simulink model "BDA_DynamicModel_v3"  (R2021b)
settings: Solver=ode23t  StartTime=0.0  StopTime=15  FixedStep=0.000001  MaxStep=1e-5  MinStep=1e-7  RelTol=1e-3
undefined symbols (not defined in the file or in its folder): X, Y, Z
libraries: sm_lib x47, nesl_utility x7
(part 3 of 5)

== matlab function BDA_DynamicModel_v3/Planta/Dinámica Directa/h ==
  data: dq1 input; h output; dq2 input; dq3 input; dq4 input; dq5 input; dq6 input; q1 input; q2 input; q3 input; q4 input; q5 input; q6 input
function h = h(dq1,dq2,dq3,dq4,dq5,dq6,q1,q2,q3,q4,q5,q6)
%#codegen

%    This function was generated by the Symbolic Math Toolbox version 9.0.
%    28-Nov-2021 14:58:02

t2 = cos(q1);
t3 = cos(q2);
t4 = cos(q4);
t5 = cos(q5);
t6 = cos(q6);
t7 = sin(q1);
t8 = sin(q2);
t9 = sin(q4);
t10 = sin(q5);
t11 = sin(q6);
t12 = dq1+dq2;
t14 = dq5.*(3.0./5.0e+2);
t22 = dq3.*5.110348748545983e-1;
t26 = dq3.*8.595599785252598e-1;
t27 = dq1.*2.038587e-2;
t28 = dq2.*2.038587e-2;
t30 = dq4.*2.889644e-2;
t31 = 9.007199254740992e+15;
t33 = dq6.*7.26735e-3;
t34 = dq5.*1.08769e-2;
t52 = dq3.*1.705747536335924e-3;
t55 = dq3.*2.869065083120968e-3;
t56 = dq3.*1.476708859914341e-2;
t58 = dq5.*6.1855407534e-5;
t59 = dq4.*6.678441185616e-4;
t60 = dq5.*1.35652563578e-4;
t61 = dq6.*1.33637554986e-4;
t62 = dq4.*1.688944904408e-4;
t63 = dq6.*7.26350557185e-5;
t65 = dq5.*7.0482312e-7;
t67 = dq4.*1.869599668e-7;
t88 = dq3.*1.749264567482926e-5;
t96 = dq3.*2.94226067152155e-5;
t97 = dq3.*1.573543573532208e-5;
t101 = dq3.*2.646698193853677e-5;
t102 = dq3.*4.515804245053758e-5;
t105 = dq3.*3.412916355515067e-4;
t106 = dq3.*8.631097478604537e-5;
t107 = dq4.*6.634286610512106e-7;
t108 = dq5.*7.314371377091851e-7;
t110 = dq6.*3.387428925624357e-6;
t111 = dq6.*1.745966317740249e-6;
t112 = dq6.*1.245668607194124e-6;
t113 = dq3.*9.554306323645785e-8;
t115 = dq5.*4.0082304082032e-9;
t116 = dq4.*2.626213073993121e-5;
t117 = dq4.*4.320951447093552e-9;
t118 = dq4.*1.092747353151976e-9;
t119 = dq5.*2.261852897508832e-6;
t120 = dq5.*5.918087154269792e-7;
t122 = dq5.*1.87902861198544e-8;
t124 = dq4.*2.3264974053944e-5;
t129 = dq3.*5.321009981904056e-7;
t135 = dq3.*4.369754608674261e-7;
t141 = dq3.*4.553682647545594e-7;
t142 = dq3.*3.390351827752591e-7;
t145 = dq3.*7.349921428868027e-7;
t153 = dq3.*1.342086469609585e-5;
t154 = dq3.*2.208156882018249e-9;
t155 = dq3.*5.584320068657135e-10;
t166 = dq3.*1.188921310415275e-5;
t13 = t12.^2;
t15 = t2.*t3.*(9.81e+2./1.0e+2);
t16 = t2.*t8.*(9.81e+2./1.0e+2);
t17 = t3.*t7.*(9.81e+2./1.0e+2);
t18 = t7.*t8.*(9.81e+2./1.0e+2);
t20 = t3.*1.051339e-1;
t21 = t8.*1.051339e-1;
t23 = t5.*5.110348748545983e-1;
t25 = t10.*5.110348748545983e-1;
t29 = t8.*3.235525e-2;
t32 = t3.*3.235525e-2;
t35 = t5.*t9.*8.595599785252598e-1;
t36 = t9.*t10.*8.595599785252598e-1;
t38 = (q3.*t31)./9.007199254740992e+15;
t41 = q3.*t31.*1.110223024625157e-16i;
t64 = t27+t28;
t68 = t2.*t8.*3.161090981652867e-3;
t69 = t3.*t7.*3.161090981652867e-3;
t70 = -t65;
t78 = t2.*t3.*4.486342129859745e-3;
t79 = t7.*t8.*4.486342129859745e-3;
t121 = -t120;
t123 = -t122;
t19 = -t18;
t24 = -t21;
t37 = -t36;
t39 = cos(t38);
t40 = sin(t38);
t42 = exp(t41);
t44 = -t41;
t66 = t20+t29;
t72 = -t68;
t73 = -t69;
t74 = t25+t35;
t80 = -t79;
t43 = t39.^2;
t45 = 1.0./t42;
t46 = t4.*t39;
t47 = t9.*t39;
t48 = t42-1.0;
t71 = t24+t32;
t75 = dq1.*dq2.*t66;
t76 = t23+t37;
t82 = t39.*1.273194e-2;
t90 = t5.*t12.*t26.*t39;
t93 = t10.*t12.*t26.*t39;
t99 = dq3.*t5.*t12.*t39.*(-8.595599785252598e-1);
t125 = t42.*3.694216783411725e-1;
t126 = t42.*1.305783216588275e-1;
t158 = t4.*t31.*t40.*5.673626844500105e-17;
t159 = t9.*t31.*t40.*5.673626844500105e-17;
t160 = t5.*t31.*t40.*9.543032792050485e-17;
t161 = t10.*t31.*t40.*9.543032792050485e-17;
t164 = t12.*t31.*t40.*5.673626844500105e-17;
t165 = t12.*t31.*t40.*9.543032792050485e-17;
t167 = t4.*t31.*t40.*3.404176106700063e-19;
t169 = t42.*3.215186923359161e-3;
t171 = t42.*1.345257168956303e-2;
t173 = t12.*t39.*t102;
t174 = dq3.*t12.*t39.*1.451749445763287e-4;
t180 = dq3.*t10.*t12.*t39.*6.243418693357491e-5;
t181 = dq3.*t10.*t12.*t39.*1.148694938939344e-4;
t183 = dq3.*t10.*t12.*t39.*5.316843277159623e-5;
t184 = dq3.*t5.*t12.*t39.*1.166015146360021e-4;
t194 = dq3.*t5.*t12.*t39.*6.058377458913066e-7;
t195 = dq3.*t10.*t12.*t39.*6.058377458913066e-7;
t196 = dq3.*t12.*t39.*1.607033050476913e-7;
t212 = t31.*t40.*4.87211480085e-18;
t215 = t12.*t31.*t40.*1.893760189037778e-19;
t220 = t4.*t31.*t40.*2.479366200131245e-18;
t221 = t12.*t31.*t40.*3.185302114428987e-19;
t225 = t12.*t31.*t40.*2.757596744935193e-18;
t226 = t4.*t31.*t40.*7.351481000981246e-18;
t227 = t9.*t31.*t40.*9.810473427588925e-18;
t228 = t9.*t31.*t40.*4.938358626738924e-18;
t240 = t12.*t39.*t129;
t241 = t12.*t39.*t141;
t242 = dq3.*t12.*t39.*(-5.321009981904056e-7);
t245 = dq3.*t12.*t39.*5.702567256462204e-7;
t246 = dq3.*t10.*t12.*t39.*3.61307032511966e-6;
t248 = dq3.*t5.*t12.*t39.*6.287140903818846e-7;
t249 = dq3.*t10.*t12.*t39.*6.287140903818846e-7;
t257 = dq3.*t12.*t39.*3.714116933072423e-9;
t260 = dq3.*t5.*t12.*t39.*3.445314443599436e-9;
t266 = dq3.*t10.*t12.*t39.*5.086950867234759e-7;
t267 = dq3.*t5.*t12.*t39.*1.944198228009988e-6;
t269 = t12.*t31.*t40.*9.963514750696585e-22;
t271 = dq3.*t12.*t39.*3.521753992522559e-6;
t273 = t12.*t31.*t40.*1.94207379898051e-21;
t274 = dq3.*t10.*t12.*t39.*1.615137793366553e-8;
t275 = t12.*t31.*t40.*1.746984305586406e-21;
t278 = t12.*t31.*t40.*3.266565541972299e-21;
t280 = t12.*t31.*t40.*2.938425274050169e-21;
t285 = t12.*t31.*t40.*1.611765660673211e-20;
t286 = t12.*t31.*t40.*6.3732583234114e-20;
t288 = t12.*t31.*t40.*1.78416509397307e-23;
t289 = t31.*t40.*t66.*5.673626844500105e-17;
t315 = t12.*t31.*t40.*7.948019859590024e-25;
t317 = t12.*t31.*t40.*2.729695842947468e-23;
t318 = t12.*t31.*t40.*4.851402178512055e-23;
t319 = t12.*t31.*t40.*8.160051999515114e-23;
t322 = t12.*t31.*t40.*6.331121467597849e-23;
t327 = t12.*t31.*t40.*2.506203748402806e-21;
t329 = t12.*t31.*t40.*4.123498135247176e-25;
t330 = t12.*t31.*t40.*1.042812382455568e-25;
t363 = t12.*t31.*t40.*2.220184103029913e-21;
t49 = t12.*t46;
t50 = t12.*t47;
t51 = t48.^2;
t53 = t47.*(3.0./5.0e+2);
t77 = dq1.*dq2.*t71;
t83 = t46.*2.228474e-2;
t84 = t47.*2.228474e-2;
t85 = t46.*6.562549e-2;
t86 = t12.*t82;
t109 = t15+t19+t75;
t127 = t45.*3.694216783411725e-1;
t128 = t45.*1.305783216588275e-1;
t130 = t13.*t43.*3.42298471896e-5;
t137 = t13.*t43.*3.07913148585e-5;
t157 = t75.*4.573233567645e-4;
t162 = -t159;
t163 = -t160;
t168 = -t164;
t170 = t45.*3.215186923359161e-3;
t172 = t45.*1.345257168956303e-2;
t176 = -t174;
t190 = -t180;
t192 = -t184;
t214 = t12.*t212;
t219 = -t215;
t229 = -t227;
t230 = -t228;
t231 = t22+t165;
t251 = -t246;
t255 = -t248;
t256 = -t249;
t261 = -t257;
t270 = t47+t158;
t276 = -t273;
t279 = -t275;
t290 = t31.*t40.*t71.*9.543032792050485e-17;
t291 = dq1.*t289;
t296 = dq1.*t31.*t40.*t71.*(-9.543032792050485e-17);
t316 = -t315;
t320 = -t318;
t321 = t52+t221;
t389 = t30+t56+t225;
t445 = t88+t278;
t446 = t102+t269;
t451 = t97+t280;
t558 = t141+t317;
t559 = t135+t319;
t561 = t62+t106+t285;
t570 = t67+t113+t288;
t54 = -t50;
t57 = t50.*(3.0./5.0e+2);
t81 = -t77;
t87 = t22.*t50;
t89 = t22.*t49;
t91 = t50.*2.889644e-2;
t92 = dq3.*t50.*(-5.110348748545983e-1);
t94 = t49.*2.228474e-2;
t95 = t50.*2.228474e-2;
t98 = t49.*2.889644e-2;
t103 = t50.*1.08769e-2;
t104 = t49.*6.562549e-2;
t131 = dq3.*t49.*2.233214539005216e-2;
t132 = t50.*6.1855407534e-5;
t133 = t49.*6.678441185616e-4;
t134 = t50.*6.678441185616e-4;
t136 = t50.*1.35652563578e-4;
t138 = dq3.*t50.*4.448078014240659e-2;
t139 = t49.*1.688944904408e-4;
t140 = t50.*1.688944904408e-4;
t146 = dq3.*t49.*2.228321578664739e-5;
t147 = t50.*7.0482312e-7;
t148 = t49.*1.869599668e-7;
t149 = t50.*1.869599668e-7;
t156 = t77.*3.222314966007e-4;
t175 = dq3.*t49.*3.161027044821787e-5;
t177 = dq3.*t49.*6.932319085178867e-5;
t178 = t50.*6.634286610512106e-7;
t179 = t50.*7.314371377091851e-7;
t182 = t50.*t106;
t185 = dq3.*t50.*4.838129975309422e-4;
t186 = dq3.*t49.*2.227142796549625e-7;
t187 = t49.*6.634286610512106e-7;
t189 = dq3.*t49.*9.866111348864255e-4;
t191 = dq3.*t50.*9.866111348864255e-4;
t199 = dq3.*t49.*4.097607071288701e-7;
t200 = t50.*4.0082304082032e-9;
t201 = t49.*t113;
t202 = t50.*2.626213073993121e-5;
t203 = t49.*4.320951447093552e-9;
t204 = t50.*4.320951447093552e-9;
t205 = t49.*1.092747353151976e-9;
t206 = t50.*1.092747353151976e-9;
t209 = t50.*2.261852897508832e-6;
t210 = t50.*5.918087154269792e-7;
t213 = t50.*1.87902861198544e-8;
t217 = t49.*4.097159105249182e-6;
t218 = t50.*4.097159105249182e-6;
t224 = t49.*2.3264974053944e-5;
t232 = dq4+t231;
t233 = t26+t168;
t247 = dq3.*t50.*6.033931856266849e-6;
t250 = dq3.*t49.*4.110811498877979e-6;
t252 = dq3.*t49.*2.048345525044518e-9;
t253 = dq3.*t50.*2.751376783138814e-6;
t254 = dq3.*t49.*1.361177298501988e-6;
t259 = dq3.*t50.*2.833525664970473e-5;
t262 = t49.*t155;
t263 = t50.*t155;
t264 = dq3.*t50.*6.383374042715173e-9;
t268 = dq3.*t49.*9.602491515741889e-9;
t272 = t46+t162;
t277 = dq3.*t49.*2.680360505776163e-5;
t281 = t6.*t270;
t282 = t11.*t270;
t292 = -t290;
t293 = dq1.*t290;
t294 = t26.*t231;
t297 = dq3.*t231.*(-8.595599785252598e-1);
t298 = t4.*t231.*1.273194e-2;
t299 = t9.*t231.*1.273194e-2;
t306 = t45.*t51.*7.997968101822611e-3;
t313 = t45.*t51.*5.407940120688672e-3;
t323 = t5.*t270.*4.334075e-2;
t324 = t10.*t270.*4.334075e-2;
t325 = t55+t219;
t326 = t31.*t40.*t109.*9.543032792050485e-17;
t332 = dq3.*t231.*1.09438660729849e-2;
t371 = t45.*t51.*t66.*2.196325630278387e-1;
t372 = t45.*t51.*t71.*2.196325630278387e-1;
t376 = dq1.*t45.*t51.*t71.*(-2.196325630278387e-1);
t377 = t31.*t40.*t109.*3.185302114428987e-19;
t380 = t96.*t231;
t382 = t101.*t231;
t385 = dq3.*t231.*(-2.646698193853677e-5);
t387 = dq3.*t231.*3.162387693460437e-4;
t430 = t45.*t51.*t109.*2.196325630278387e-1;
t447 = t96+t276;
t448 = t31.*t40.*t109.*3.266565541972299e-21;
t450 = t31.*t40.*t109.*2.938425274050169e-21;
t454 = t101+t279;
t456 = t145.*t231;
t460 = dq3.*t231.*1.848358683849143e-6;
t462 = t125+t127+2.61156643317655e-1;
t463 = t126+t128+7.38843356682345e-1;
t464 = dq3.*t231.*2.046064837668903e-9;
t482 = t45.*t51.*t109.*7.330961578512107e-4;
t498 = t12.*t39.*t231.*4.610311905110107e-7;
t499 = t12.*t39.*t231.*2.657686288317005e-7;
t516 = t45.*t51.*t109.*6.762775401369527e-6;
t555 = t12.*t39.*t446;
t557 = t129+t316;
t560 = t145+t320;
t577 = t12.*t39.*t559;
t612 = t231.*t445;
t692 = t214+t291+t296;
t100 = -t91;
t114 = t16+t17+t81;
t143 = -t134;
t144 = -t140;
t150 = -t147;
t151 = -t148;
t152 = -t149;
t188 = -t178;
t193 = -t185;
t197 = -t189;
t198 = -t191;
t207 = -t203;
t208 = -t204;
t211 = -t210;
t216 = -t213;
t222 = -t217;
t223 = -t218;
t234 = t5.*t232;
t235 = t10.*t232;
t236 = t4.*t233;
t237 = t9.*t233;
t258 = -t253;
t265 = -t264;
t283 = t5.*t272;
t284 = t10.*t272;
t287 = -t282;
t295 = t22.*t233;
t300 = -t299;
t334 = dq3.*t233.*6.506465364556255e-3;
t373 = dq1.*t371;
t374 = -t372;
t375 = dq1.*t372;
t381 = t88.*t233;
t383 = t97.*t233;
t384 = dq3.*t233.*(-1.749264567482926e-5);
t386 = dq3.*t233.*1.880136860189779e-4;
t433 = -t430;
t452 = -t448;
t457 = t135.*t233;
t458 = dq3.*t233.*1.098906152317443e-6;
t459 = dq3.*t233.*(-4.369754608674261e-7);
t465 = dq3.*t233.*1.216448548542787e-9;
t500 = t12.*t39.*t233.*2.657686288317005e-7;
t501 = t12.*t39.*t233.*4.440483400039196e-7;
t520 = -t516;
t556 = -t555;
t565 = t66.*t463;
t566 = t71.*t462;
t573 = t109.*t462;
t578 = t12.*t39.*t560;
t579 = -t577;
t614 = t231.*t447;
t616 = t233.*t451;
t617 = t233.*t454;
t676 = t231.*t557;
t680 = t233.*t558;
t681 = t232.*t561;
t684 = t232.*t570;
t689 = t212+t289+t292;
t694 = t4.*t692;
t695 = t9.*t692;
t697 = t169+t170+t306+1.819229615328168e-2;
t698 = t171+t172+t313+9.510076620873934e-3;
t706 = t22.*t692;
t709 = t26.*t692;
t711 = t52.*t692;
t712 = dq3.*t692.*(-1.705747536335924e-3);
t713 = t55.*t692;
t714 = dq3.*t692.*2.483822334585646e-2;
t717 = t102.*t692;
t719 = dq3.*t692.*1.451749445763287e-4;
t722 = dq3.*t692.*1.607033050476913e-7;
t727 = t12.*t39.*t692.*3.42298471896e-5;
t728 = t12.*t39.*t692.*3.07913148585e-5;
t753 = t321.*t692;
t754 = t325.*t692;
t798 = t446.*t692;
t238 = -t234;
t239 = -t236;
t243 = t236.*(3.0./5.0e+2);
t301 = t236.*2.889644e-2;
t302 = t234.*1.08769e-2;
t303 = t237.*2.889644e-2;
t304 = t235.*1.08769e-2;
t305 = t236.*2.228474e-2;
t307 = t237.*2.228474e-2;
t308 = t235.*7.26735e-3;
t309 = t237.*6.562549e-2;
t312 = t236.*1.08769e-2;
t328 = t31.*t40.*t114.*5.673626844500105e-17;
t333 = t49+t237;
t335 = -t334;
t336 = t54+t236;
t337 = t234.*1.35652563578e-4;
t338 = t235.*1.35652563578e-4;
t339 = t235.*1.33637554986e-4;
t340 = t234.*6.1855407534e-5;
t341 = t235.*7.26350557185e-5;
t342 = t235.*6.1855407534e-5;
t344 = t237.*1.688944904408e-4;
t345 = t236.*6.1855407534e-5;
t350 = t236.*6.678441185616e-4;
t351 = t237.*6.678441185616e-4;
t353 = t236.*1.35652563578e-4;
t354 = t236.*1.688944904408e-4;
t355 = t234.*7.0482312e-7;
t356 = t235.*7.0482312e-7;
t362 = t236.*7.0482312e-7;
t364 = t236.*1.869599668e-7;
t365 = t237.*1.869599668e-7;
t378 = t31.*t40.*t114.*1.893760189037778e-19;
t388 = -t386;
t390 = t234.*7.314371377091851e-7;
t391 = t235.*7.314371377091851e-7;
t392 = t236.*6.634286610512106e-7;
t393 = t237.*6.634286610512106e-7;
t394 = t236.*7.314371377091851e-7;
t395 = t235.*3.387428925624357e-6;
t396 = t234.*2.663570267859459e-6;
t397 = t235.*2.663570267859459e-6;
t398 = t235.*1.745966317740249e-6;
t399 = t235.*1.245668607194124e-6;
t400 = t234.*4.0082304082032e-9;
t401 = t235.*4.0082304082032e-9;
t405 = t236.*4.0082304082032e-9;
t410 = t236.*2.626213073993121e-5;
t412 = t236.*1.092747353151976e-9;
t413 = t237.*1.092747353151976e-9;
t416 = t236.*4.320951447093552e-9;
t417 = t237.*4.320951447093552e-9;
t428 = t234.*5.918087154269792e-7;
t429 = t235.*2.261852897508832e-6;
t432 = t236.*2.261852897508832e-6;
t434 = t236.*5.918087154269792e-7;
t436 = t45.*t51.*t114.*2.196325630278387e-1;
t437 = t234.*1.87902861198544e-8;
t438 = t235.*1.87902861198544e-8;
t439 = t236.*1.87902861198544e-8;
t441 = t236.*4.097159105249182e-6;
t442 = t237.*4.097159105249182e-6;
t443 = t237.*2.3264974053944e-5;
t449 = t31.*t40.*t114.*1.94207379898051e-21;
t453 = t31.*t40.*t114.*1.746984305586406e-21;
t461 = -t458;
t466 = -t465;
t490 = t45.*t51.*t114.*7.330961578512107e-4;
t497 = t45.*t51.*t114.*6.346599179580158e-3;
t502 = -t500;
t503 = -t501;
t519 = t45.*t51.*t114.*7.517989070303108e-6;
t526 = t161+t283;
t533 = t163+t284;
t540 = t45.*t51.*t114.*3.70947298167937e-5;
t545 = -t6.*(t160-t284);
t546 = -t11.*(t160-t284);
t547 = t45.*t51.*t114.*4.106249669188362e-8;
t567 = dq1.*t565;
t568 = dq1.*t566;
t569 = -t566;
t574 = t114.*t463;
t575 = -t573;
t576 = t295+t297;
t580 = -t4.*(t294-t295);
t581 = -t9.*(t294-t295);
t592 = t573.*3.33783e-3;
t593 = t573.*2.889644e-2;
t600 = t9.*(t294-t295).*(-2.228474e-2);
t601 = t4.*(t294-t295).*(-6.562549e-2);
t602 = t4.*(t294-t295).*6.562549e-2;
t603 = t9.*(t294-t295).*(-4.36041e-5);
t606 = t573.*3.42298471896e-5;
t609 = t573.*1.688944904408e-4;
t611 = t573.*1.869599668e-7;
t615 = -t614;
t618 = -t616;
t619 = t4.*(t294-t295).*(-1.3117937708872e-3);
t620 = t9.*(t294-t295).*(-1.3117937708872e-3);
t621 = t9.*(t294-t295).*(-1.35652563578e-4);
h = ft_1({dq1,dq2,dq3,dq4,dq5,dq6,t10,t100,t101,t103,t104,t105,t107,t108,t109,t11,t110,t111,t112,t114,t115,t116,t117,t118,t119,t12,t120,t121,t122,t123,t124,t130,t131,t132,t133,t134,t136,t137,t138,t139,t14,t140,t142,t143,t144,t146,t147,t148,t149,t150,t151,t152,t153,t154,t155,t156,t157,t160,t166,t167,t173,t174,t175,t176,t177,t179,t181,t182,t183,t184,t185,t186,t187,t188,t189,t190,t191,t192,t193,t194,t195,t196,t197,t198,t199,t2,t200,t201,t202,t204,t205,t206,t207,t208,t209,t211,t212,t216,t22,t220,t222,t223,t224,t226,t229,t230,t231,t232,t233,t234,t235,t238,t239,t241,t242,t243,t245,t246,t247,t250,t251,t252,t254,t255,t256,t258,t259,t26,t260,t261,t262,t263,t265,t266,t267,t268,t270,t271,t272,t274,t277,t281,t282,t284,t286,t287,t294,t295,t298,t3,t30,t300,t301,t302,t303,t304,t305,t307,t308,t309,t31,t312,t321,t322,t323,t324,t325,t326,t327,t328,t329,t33,t330,t332,t333,t335,t337,t338,t339,t34,t340,t341,t342,t344,t345,t350,t351,t353,t354,t355,t356,t362,t363,t364,t365,t371,t373,t374,t376,t377,t378,t380,t383,t384,t385,t387,t388,t389,t39,t390,t391,t392,t393,t394,t395,t396,t397,t398,t399,t4,t40,t400,t401,t405,t410,t412,t413,t416,t417,t428,t429,t432,t433,t434,t436,t437,t438,t439,t441,t442,t443,t445,t447,t449,t450,t451,t452,t453,t454,t456,t459,t460,t461,t464,t466,t482,t49,t490,t497,t498,t499,t5,t50,t502,t503,t519,t52,t520,t526,t53,t540,t545,t546,t547,t55,t556,t561,t565,t567,t568,t569,t57,t570,t574,t575,t577,t578,t579,t58,t580,t581,t59,t592,t593,t6,t60,t600,t602,t603,t606,t609,t61,t611,t612,t615,t617,t618,t619,t62,t620,t621,t63,t64,t65,t66,t67,t676,t680,t681,t684,t689,t692,t694,t695,t697,t698,t7,t70,t706,t709,t71,t712,t713,t714,t717,t719,t72,t722,t727,t728,t73,t74,t75,t753,t754,t76,t77,t78,t798,t8,t80,t82,t83,t84,t85,t86,t88,t89,t9,t90,t91,t92,t93,t94,t95,t96,t97,t98,t99});
end
function h = ft_1(ct)
dq1 = ct{1};
dq2 = ct{2};
dq3 = ct{3};
dq4 = ct{4};
dq5 = ct{5};
dq6 = ct{6};
t10 = ct{7};
t100 = ct{8};
t101 = ct{9};
t103 = ct{10};
t104 = ct{11};
t105 = ct{12};
t107 = ct{13};
t108 = ct{14};
t109 = ct{15};
t11 = ct{16};
t110 = ct{17};
t111 = ct{18};
t112 = ct{19};
t114 = ct{20};
t115 = ct{21};
t116 = ct{22};
t117 = ct{23};
t118 = ct{24};
t119 = ct{25};
t12 = ct{26};
t120 = ct{27};
t121 = ct{28};
t122 = ct{29};
t123 = ct{30};
t124 = ct{31};
t130 = ct{32};
t131 = ct{33};
t132 = ct{34};
t133 = ct{35};
t134 = ct{36};
t136 = ct{37};
t137 = ct{38};
t138 = ct{39};
t139 = ct{40};
t14 = ct{41};
t140 = ct{42};
t142 = ct{43};
t143 = ct{44};
t144 = ct{45};
t146 = ct{46};
t147 = ct{47};
t148 = ct{48};
t149 = ct{49};
t150 = ct{50};
t151 = ct{51};
t152 = ct{52};
t153 = ct{53};
t154 = ct{54};
t155 = ct{55};
t156 = ct{56};
t157 = ct{57};
t160 = ct{58};
t166 = ct{59};
t167 = ct{60};
t173 = ct{61};
t174 = ct{62};
t175 = ct{63};
t176 = ct{64};
t177 = ct{65};
t179 = ct{66};
t181 = ct{67};
t182 = ct{68};
t183 = ct{69};
t184 = ct{70};
t185 = ct{71};
t186 = ct{72};
t187 = ct{73};
t188 = ct{74};
t189 = ct{75};
t190 = ct{76};
t191 = ct{77};
t192 = ct{78};
t193 = ct{79};
t194 = ct{80};
t195 = ct{81};
t196 = ct{82};
t197 = ct{83};
t198 = ct{84};
t199 = ct{85};
t2 = ct{86};
t200 = ct{87};
t201 = ct{88};
t202 = ct{89};
t204 = ct{90};
t205 = ct{91};
t206 = ct{92};
t207 = ct{93};
t208 = ct{94};
t209 = ct{95};
t211 = ct{96};
t212 = ct{97};
t216 = ct{98};
t22 = ct{99};
t220 = ct{100};
t222 = ct{101};
t223 = ct{102};
t224 = ct{103};
t226 = ct{104};
t229 = ct{105};
t230 = ct{106};
t231 = ct{107};
t232 = ct{108};
t233 = ct{109};
t234 = ct{110};
t235 = ct{111};
t238 = ct{112};
t239 = ct{113};
t241 = ct{114};
t242 = ct{115};
t243 = ct{116};
t245 = ct{117};
t246 = ct{118};
t247 = ct{119};
t250 = ct{120};
t251 = ct{121};
t252 = ct{122};
t254 = ct{123};
t255 = ct{124};
t256 = ct{125};
t258 = ct{126};
t259 = ct{127};
t26 = ct{128};
t260 = ct{129};
t261 = ct{130};
t262 = ct{131};
t263 = ct{132};
t265 = ct{133};
t266 = ct{134};
t267 = ct{135};
t268 = ct{136};
t270 = ct{137};
t271 = ct{138};
t272 = ct{139};
t274 = ct{140};
t277 = ct{141};
t281 = ct{142};
t282 = ct{143};
t284 = ct{144};
t286 = ct{145};
t287 = ct{146};
t294 = ct{147};
t295 = ct{148};
t298 = ct{149};
t3 = ct{150};
t30 = ct{151};
t300 = ct{152};
t301 = ct{153};
t302 = ct{154};
t303 = ct{155};
t304 = ct{156};
t305 = ct{157};
t307 = ct{158};
t308 = ct{159};
t309 = ct{160};
t31 = ct{161};
t312 = ct{162};
t321 = ct{163};
t322 = ct{164};
t323 = ct{165};
t324 = ct{166};
t325 = ct{167};
t326 = ct{168};
t327 = ct{169};
t328 = ct{170};
t329 = ct{171};
t33 = ct{172};
t330 = ct{173};
t332 = ct{174};
t333 = ct{175};
t335 = ct{176};
t337 = ct{177};
t338 = ct{178};
t339 = ct{179};
t34 = ct{180};
t340 = ct{181};
t341 = ct{182};
t342 = ct{183};
t344 = ct{184};
t345 = ct{185};
t350 = ct{186};
t351 = ct{187};
t353 = ct{188};
t354 = ct{189};
t355 = ct{190};
t356 = ct{191};
t362 = ct{192};
t363 = ct{193};
t364 = ct{194};
t365 = ct{195};
t371 = ct{196};
t373 = ct{197};
t374 = ct{198};
t376 = ct{199};
t377 = ct{200};
t378 = ct{201};
t380 = ct{202};
t383 = ct{203};
t384 = ct{204};
t385 = ct{205};
t387 = ct{206};
t388 = ct{207};
t389 = ct{208};
t39 = ct{209};
t390 = ct{210};
t391 = ct{211};
t392 = ct{212};
t393 = ct{213};
t394 = ct{214};
t395 = ct{215};
t396 = ct{216};
t397 = ct{217};
t398 = ct{218};
t399 = ct{219};
t4 = ct{220};
t40 = ct{221};
t400 = ct{222};
t401 = ct{223};
t405 = ct{224};
t410 = ct{225};
t412 = ct{226};
t413 = ct{227};
t416 = ct{228};
t417 = ct{229};
t428 = ct{230};
t429 = ct{231};
t432 = ct{232};
t433 = ct{233};
t434 = ct{234};
t436 = ct{235};
t437 = ct{236};
t438 = ct{237};
t439 = ct{238};
t441 = ct{239};
t442 = ct{240};
t443 = ct{241};
t445 = ct{242};
t447 = ct{243};
t449 = ct{244};
t450 = ct{245};
t451 = ct{246};
t452 = ct{247};
t453 = ct{248};
t454 = ct{249};
t456 = ct{250};
t459 = ct{251};
t460 = ct{252};
t461 = ct{253};
t464 = ct{254};
t466 = ct{255};
t482 = ct{256};
t49 = ct{257};
t490 = ct{258};
t497 = ct{259};
t498 = ct{260};
t499 = ct{261};
t5 = ct{262};
t50 = ct{263};
t502 = ct{264};
t503 = ct{265};
t519 = ct{266};
t52 = ct{267};
t520 = ct{268};
t526 = ct{269};
t53 = ct{270};
t540 = ct{271};
t545 = ct{272};
t546 = ct{273};
t547 = ct{274};
t55 = ct{275};
t556 = ct{276};
t561 = ct{277};
t565 = ct{278};
t567 = ct{279};
t568 = ct{280};
t569 = ct{281};
t57 = ct{282};
t570 = ct{283};
t574 = ct{284};
t575 = ct{285};
t577 = ct{286};
t578 = ct{287};
t579 = ct{288};
t58 = ct{289};
t580 = ct{290};
t581 = ct{291};
t59 = ct{292};
t592 = ct{293};
t593 = ct{294};
t6 = ct{295};
t60 = ct{296};
t600 = ct{297};
t602 = ct{298};
t603 = ct{299};
t606 = ct{300};
t609 = ct{301};
t61 = ct{302};
t611 = ct{303};
t612 = ct{304};
t615 = ct{305};
t617 = ct{306};
t618 = ct{307};
t619 = ct{308};
t62 = ct{309};
t620 = ct{310};
t621 = ct{311};
t63 = ct{312};
t64 = ct{313};
t65 = ct{314};
t66 = ct{315};
t67 = ct{316};
t676 = ct{317};
t680 = ct{318};
t681 = ct{319};
t684 = ct{320};
t689 = ct{321};
t692 = ct{322};
t694 = ct{323};
t695 = ct{324};
t697 = ct{325};
t698 = ct{326};
t7 = ct{327};
t70 = ct{328};
t706 = ct{329};
t709 = ct{330};
t71 = ct{331};
t712 = ct{332};
t713 = ct{333};
t714 = ct{334};
t717 = ct{335};
t719 = ct{336};
t72 = ct{337};
t722 = ct{338};
t727 = ct{339};
t728 = ct{340};
t73 = ct{341};
t74 = ct{342};
t75 = ct{343};
t753 = ct{344};
t754 = ct{345};
t76 = ct{346};
t77 = ct{347};
t78 = ct{348};
t798 = ct{349};
t8 = ct{350};
t80 = ct{351};
t82 = ct{352};
t83 = ct{353};
t84 = ct{354};
t85 = ct{355};
t86 = ct{356};
t88 = ct{357};
t89 = ct{358};
t9 = ct{359};
t90 = ct{360};
t91 = ct{361};
t92 = ct{362};
t93 = ct{363};
t94 = ct{364};
t95 = ct{365};
t96 = ct{366};
t97 = ct{367};
t98 = ct{368};
t99 = ct{369};
t622 = t4.*(t294-t295).*(-1.688944904408e-4);
t623 = t9.*(t294-t295).*1.3117937708872e-3;
t624 = t9.*(t294-t295).*(-6.1855407534e-5);
t625 = t4.*(t294-t295).*1.688944904408e-4;
t626 = t9.*(t294-t295).*(-4.35810334311e-7);
t627 = t4.*(t294-t295).*(-7.13801892181e-4);
t628 = t9.*(t294-t295).*(-1.869599668e-7);
t630 = t9.*(t294-t295).*(-8.01825329916e-7);
t646 = t4.*(t294-t295).*(-8.902265954562403e-6);
t647 = t9.*(t294-t295).*(-4.427198467956924e-6);
t648 = t9.*(t294-t295).*(-2.663570267859459e-6);
t649 = t4.*(t294-t295).*(-4.059291428568442e-6);
t650 = t4.*(t294-t295).*8.902265954562403e-6;
t651 = t9.*(t294-t295).*(-4.0082304082032e-9);
t653 = t4.*(t294-t295).*(-4.114486328260564e-5);
t654 = t4.*(t294-t295).*(-8.487305697640184e-9);
t655 = t4.*(t294-t295).*(-1.092747353151976e-9);
t656 = t9.*(t294-t295).*(-1.092747353151976e-9);
t657 = t4.*(t294-t295).*4.114486328260564e-5;
t660 = t4.*(t294-t295).*1.092747353151976e-9;
t674 = t9.*(t294-t295).*(-1.87902861198544e-8);
t675 = t9.*(t294-t295).*(-3.814770659661843e-5);
t677 = -t676;
t690 = t4.*t689;
t691 = t9.*t689;
t696 = -t695;
t699 = t4.*t697;
t700 = t9.*t697;
t701 = t12.*t697;
t702 = t12.*t698;
t723 = t82+t698;
t755 = -t754;
t799 = -t798;
t841 = t374+t565+t697;
t244 = -t243;
t310 = -t302;
t311 = -t305;
t314 = -t312;
t331 = -t328;
t343 = dq4.*t333;
t346 = -t337;
t347 = t5.*t333;
t348 = t10.*t333;
t349 = dq5+t50+t239;
t352 = -t340;
t357 = -t345;
t358 = -t353;
t359 = -dq4.*(t50+t239);
t360 = -t354;
t361 = -t355;
t366 = -t362;
t369 = -t365;
t379 = -t378;
t402 = -t394;
t403 = -t396;
t404 = -t400;
t408 = -t405;
t411 = dq4.*(t50+t239).*(-4.334075e-2);
t414 = t5.*(t50+t239).*(-4.334075e-2);
t415 = t10.*(t50+t239).*(-4.334075e-2);
t418 = -t410;
t419 = dq4.*(t50+t239).*4.334075e-2;
t421 = -t412;
t422 = t5.*(t50+t239).*4.334075e-2;
t423 = t10.*(t50+t239).*4.334075e-2;
t424 = -t416;
t425 = -t417;
t435 = -t432;
t440 = -t437;
t444 = -t442;
t455 = -t453;
t467 = t98+t303;
t469 = t59.*t333;
t470 = t100+t301;
t479 = dq4.*(t50+t239).*(-4.71413003675e-4);
t481 = dq4.*(t50+t239).*(-6.678441185616e-4);
t484 = dq4.*(t50+t239).*(-1.688944904408e-4);
t485 = t67.*t333;
t486 = t62.*(t50+t239);
t504 = t107.*t333;
t508 = dq4.*(t50+t239).*(-5.879283844893203e-6);
t509 = dq4.*(t50+t239).*(-2.68085975407921e-6);
t518 = dq4.*(t50+t239).*5.879283844893203e-6;
t525 = t118.*t333;
t527 = dq4.*(t50+t239).*(-2.626213073993121e-5);
t534 = dq4.*(t50+t239).*(-4.320951447093552e-9);
t535 = t116.*(t50+t239);
t538 = dq4.*(t50+t239).*(-1.092747353151976e-9);
t541 = t118.*(t50+t239);
t549 = t6.*t526.*(3.0./5.0e+2);
t550 = t11.*t526.*(3.0./5.0e+2);
t553 = t124.*t333;
t562 = t133+t351;
t563 = t139+t344;
t564 = t143+t350;
t571 = t152+t364;
t572 = -t568;
t594 = -t592;
t595 = -t593;
t596 = t574.*3.33783e-3;
t607 = -t606;
t608 = t574.*3.07913148585e-5;
t610 = -t609;
t613 = -t611;
t682 = t281+t546;
t683 = t287+t545;
t693 = -t691;
t705 = (t50+t239).*(t134-t350);
t710 = (t50+t239).*(t149-t364);
t724 = t10.*t723;
t725 = t5.*t723;
t732 = t59+t105+t144+t286+t354;
t741 = -t5.*(dq4.*(t50+t239)+dq3.*t50.*5.110348748545983e-1+t4.*(t294-t295));
t742 = -t10.*(dq4.*(t50+t239)+dq3.*t50.*5.110348748545983e-1+t4.*(t294-t295));
t761 = t5.*(dq4.*(t50+t239)+dq3.*t50.*5.110348748545983e-1+t4.*(t294-t295)).*(-7.26350557185e-5);
t762 = t5.*(dq4.*(t50+t239)+dq3.*t50.*5.110348748545983e-1+t4.*(t294-t295)).*(-6.1855407534e-5);
t763 = t10.*(dq4.*(t50+t239)+dq3.*t50.*5.110348748545983e-1+t4.*(t294-t295)).*(-1.35652563578e-4);
t764 = t5.*(dq4.*(t50+t239)+dq3.*t50.*5.110348748545983e-1+t4.*(t294-t295)).*(-1.33637554986e-4);
t765 = t5.*(dq4.*(t50+t239)+dq3.*t50.*5.110348748545983e-1+t4.*(t294-t295)).*7.26350557185e-5;
t766 = t5.*(dq4.*(t50+t239)+dq3.*t50.*5.110348748545983e-1+t4.*(t294-t295)).*(-7.0482312e-7);
t767 = t10.*(dq4.*(t50+t239)+dq3.*t50.*5.110348748545983e-1+t4.*(t294-t295)).*(-7.0482312e-7);
t768 = t10.*(dq4.*(t50+t239)+dq3.*t50.*5.110348748545983e-1+t4.*(t294-t295)).*7.0482312e-7;
t779 = t5.*(dq4.*(t50+t239)+dq3.*t50.*5.110348748545983e-1+t4.*(t294-t295)).*(-7.314371377091851e-7);
t780 = t10.*(dq4.*(t50+t239)+dq3.*t50.*5.110348748545983e-1+t4.*(t294-t295)).*(-7.314371377091851e-7);
t781 = t5.*(dq4.*(t50+t239)+dq3.*t50.*5.110348748545983e-1+t4.*(t294-t295)).*(-4.203395243364607e-6);
t782 = t5.*(dq4.*(t50+t239)+dq3.*t50.*5.110348748545983e-1+t4.*(t294-t295)).*7.314371377091851e-7;
t783 = t5.*(dq4.*(t50+t239)+dq3.*t50.*5.110348748545983e-1+t4.*(t294-t295)).*4.203395243364607e-6;
t784 = t10.*(dq4.*(t50+t239)+dq3.*t50.*5.110348748545983e-1+t4.*(t294-t295)).*(-4.0082304082032e-9);
t785 = t10.*(dq4.*(t50+t239)+dq3.*t50.*5.110348748545983e-1+t4.*(t294-t295)).*4.0082304082032e-9;
t787 = t10.*(dq4.*(t50+t239)+dq3.*t50.*5.110348748545983e-1+t4.*(t294-t295)).*(-2.261852897508832e-6);
t788 = t5.*(dq4.*(t50+t239)+dq3.*t50.*5.110348748545983e-1+t4.*(t294-t295)).*(-5.918087154269792e-7);
t790 = t10.*(dq4.*(t50+t239)+dq3.*t50.*5.110348748545983e-1+t4.*(t294-t295)).*2.261852897508832e-6;
t791 = t84+t226+t700;
t792 = t5.*(dq4.*(t50+t239)+dq3.*t50.*5.110348748545983e-1+t4.*(t294-t295)).*(-1.87902861198544e-8);
t793 = t187+t208+t393+t416;
t794 = t85+t229+t699;
t801 = t118+t155+t187+t330+t393;
t804 = t107+t142+t223+t322+t441;
t807 = t124+t166+t188+t363+t392;
t842 = t4.*t841;
t843 = t9.*t841;
t844 = t376+t567+t701;
t859 = t433+t574+t706;
t863 = t371+t569+t723;
t958 = t332+t335+t436+t575+t709;
t367 = t6.*t349;
t368 = t11.*t349;
t406 = t347.*1.08769e-2;
t407 = t348.*1.08769e-2;
t409 = t347.*7.26735e-3;
t420 = t343.*4.36041e-5;
t468 = t343.*6.1855407534e-5;
t471 = t343.*1.35652563578e-4;
t472 = t347.*1.35652563578e-4;
t473 = t348.*1.35652563578e-4;
t474 = t347.*1.33637554986e-4;
t475 = t343.*(-6.678441185616e-4);
t476 = t347.*7.26350557185e-5;
t477 = t347.*6.1855407534e-5;
t478 = t348.*6.1855407534e-5;
t480 = t343.*4.35810334311e-7;
t487 = t347.*7.0482312e-7;
t488 = t348.*7.0482312e-7;
t489 = t343.*8.01825329916e-7;
t505 = t347.*7.314371377091851e-7;
t506 = t348.*7.314371377091851e-7;
t507 = t343.*2.663570267859459e-6;
t510 = t347.*3.387428925624357e-6;
t511 = t347.*2.663570267859459e-6;
t512 = t348.*2.663570267859459e-6;
t513 = t347.*1.745966317740249e-6;
t514 = t347.*1.245668607194124e-6;
t515 = t343.*4.0082304082032e-9;
t521 = t347.*4.0082304082032e-9;
t522 = t348.*4.0082304082032e-9;
t539 = t34+t103+t314;
t542 = t348.*5.918087154269792e-7;
t543 = t347.*2.261852897508832e-6;
t548 = t343.*1.87902861198544e-8;
t551 = t347.*1.87902861198544e-8;
t552 = t348.*1.87902861198544e-8;
t582 = t235+t347;
t584 = t238+t348;
t586 = -dq5.*(t234-t348);
t587 = -t6.*(t234-t348);
t588 = -t11.*(t234-t348);
t589 = dq5.*(t234-t348);
t597 = -t596;
t598 = t60+t136+t358;
t599 = t58+t132+t357;
t604 = t6.*(t234-t348).*(-7.26735e-3);
t605 = t11.*(t234-t348).*(-7.26735e-3);
t637 = t58.*(t234-t348);
t638 = t6.*(t234-t348).*(-1.33637554986e-4);
t639 = t11.*(t234-t348).*(-1.33637554986e-4);
t640 = t6.*(t234-t348).*(-7.26350557185e-5);
t642 = t11.*(t234-t348).*(-7.26350557185e-5);
t645 = t65.*(t234-t348);
t662 = t6.*(t234-t348).*(-4.203395243364607e-6);
t663 = t11.*(t234-t348).*(-4.203395243364607e-6);
t665 = t6.*(t234-t348).*(-3.387428925624357e-6);
t666 = t6.*(t234-t348).*(-1.245668607194124e-6);
t667 = t11.*(t234-t348).*(-1.745966317740249e-6);
t668 = t11.*(t234-t348).*(-1.245668607194124e-6);
t673 = t120.*(t234-t348);
t679 = t122.*(t234-t348);
t703 = t333.*t562;
t704 = t333.*t563;
t726 = -t724;
t736 = t59+t105+t151+t286+t369;
t738 = t140+t148+t360+t365;
t739 = t89+t343+t581;
t740 = t92+t359+t580;
t795 = t5.*t791;
t796 = t10.*t791;
t797 = t202+t205+t413+t418;
t800 = t206+t224+t421+t443;
t802 = t116+t153+t207+t327+t425;
t803 = t118+t155+t204+t330+t424;
t806 = t117+t154+t222+t329+t444;
t811 = t333.*t732;
t820 = t232.*t793;
t822 = t232.*t804;
t829 = -t801.*(t50+t239);
t831 = t801.*(t50+t239);
t838 = -t807.*(t50+t239);
t845 = t373+t572+t702;
t846 = t4.*t844;
t847 = t9.*t844;
t851 = t22.*t844;
t857 = t52.*t844;
t860 = t4.*t859;
t861 = t9.*t859;
t864 = t5.*t863;
t865 = t10.*t863;
t870 = t12.*t39.*t844.*3.33783e-3;
t872 = t88.*t844;
t873 = t97.*t844;
t874 = dq3.*t844.*(-1.749264567482926e-5);
t924 = t321.*t844;
t935 = t451.*t844;
t937 = t454.*t844;
t959 = t5.*t958;
t961 = t10.*t958.*7.26735e-3;
t963 = t10.*t958.*1.08769e-2;
t965 = t10.*t958.*7.26350557185e-5;
t966 = t10.*t958.*6.1855407534e-5;
t968 = t10.*t958.*1.33637554986e-4;
t971 = t10.*t958.*7.0482312e-7;
t975 = t84+t220+t690+t843;
t978 = t85+t230+t693+t842;
t1085 = t456+t459+t519+t520+t607+t608+t677+t680+t717+t799;
t370 = -t368;
t426 = t367.*7.26735e-3;
t427 = t368.*7.26735e-3;
t483 = -t478;
t491 = t367.*1.33637554986e-4;
t492 = t368.*1.33637554986e-4;
t493 = t367.*7.26350557185e-5;
t494 = t368.*7.26350557185e-5;
t517 = -t506;
t523 = t367.*4.203395243364607e-6;
t524 = t368.*4.203395243364607e-6;
t528 = t368.*3.387428925624357e-6;
t530 = t367.*1.745966317740249e-6;
t531 = t367.*1.245668607194124e-6;
t532 = t368.*1.245668607194124e-6;
t544 = -t542;
t554 = -t552;
t583 = dq6+t582;
t585 = dq5.*t582;
t590 = t6.*t582.*(3.0./5.0e+2);
t591 = t11.*t582.*(3.0./5.0e+2);
t629 = t60.*t582;
t631 = t304+t406;
t632 = t589.*(-7.26350557185e-5);
t633 = t589.*(-6.1855407534e-5);
t634 = t65.*t582;
t635 = t310+t407;
t636 = t589.*(-1.33637554986e-4);
t643 = t589.*1.33637554986e-4;
t644 = t589.*(-7.0482312e-7);
t652 = t108.*t582;
t658 = t589.*(-7.314371377091851e-7);
t659 = t115.*t582;
t661 = t589.*(-4.203395243364607e-6);
t669 = t33+t308+t409;
t670 = t119.*t582;
t672 = t589.*(-5.918087154269792e-7);
t678 = t589.*(-1.87902861198544e-8);
t685 = t342+t477;
t686 = t346+t473;
t687 = t356+t487;
t688 = t361+t488;
t707 = t63+t341+t476;
t708 = t61+t339+t474;
t715 = t367+t588;
t718 = t349.*t599;
t720 = t349.*t598;
t729 = t111+t398+t513;
t730 = t112+t399+t514;
t731 = t110+t395+t510;
t737 = dq6.*(t368+t6.*(t234-t348)).*(-1.33637554986e-4);
t745 = dq6.*(t368+t6.*(t234-t348)).*(-1.245668607194124e-6);
t746 = dq6.*(t368+t6.*(t234-t348)).*(-3.387428925624357e-6);
t747 = t10.*t739.*4.334075e-2;
t756 = t5.*t739.*4.71413003675e-4;
t757 = t10.*t739.*4.71413003675e-4;
t758 = t5.*t739.*3.149723995125e-4;
t759 = t11.*t739.*7.26350557185e-5;
t760 = t6.*t739.*1.33637554986e-4;
t769 = t5.*t739.*2.68085975407921e-6;
t770 = t5.*t739.*3.148057791131579e-6;
t771 = t10.*t739.*5.879283844893203e-6;
t772 = t5.*t739.*5.791951861259479e-6;
t773 = t6.*t739.*1.245668607194124e-6;
t774 = t11.*t739.*1.745966317740249e-6;
t775 = t11.*t739.*1.245668607194124e-6;
t776 = t5.*t739.*3.054756263814e-8;
t777 = t10.*t739.*3.054756263814e-8;
t778 = t6.*t739.*3.387428925624357e-6;
t805 = t232.*t738;
t810 = (t234-t348).*(t337-t473);
t814 = -t736.*(t50+t239);
t815 = t736.*(t50+t239);
t816 = t65+t147+t352+t366+t478;
t817 = t70+t150+t338+t362+t472;
t821 = -t820;
t823 = -t822;
t825 = t232.*t806;
t827 = t333.*t797;
t828 = -t800.*(t50+t239);
t830 = t108+t179+t401+t402+t521;
t832 = t333.*t802;
t833 = t115+t200+t403+t408+t512;
t835 = t333.*t803;
t836 = t119+t209+t404+t435+t522;
t839 = t123+t216+t397+t439+t511;
t840 = t121+t211+t434+t438+t551;
t850 = t401+t440+t521+t552;
t852 = t26.*t845;
t854 = t93+t589+t741;
t858 = t55.*t845;
t862 = -t861;
t866 = -t865;
t871 = t12.*t39.*t845.*3.33783e-3;
t875 = t86+t845;
t876 = t96.*t845;
t878 = t101.*t845;
t880 = dq3.*t845.*(-2.94226067152155e-5);
t882 = t860.*2.889644e-2;
t883 = t861.*2.889644e-2;
t884 = t860.*1.08769e-2;
t895 = t860.*1.35652563578e-4;
t896 = t861.*1.688944904408e-4;
t897 = t860.*6.1855407534e-5;
t898 = t860.*6.678441185616e-4;
t899 = t861.*6.678441185616e-4;
t903 = t860.*1.869599668e-7;
t925 = -t924;
t926 = t325.*t845;
t936 = t445.*t845;
t938 = t447.*t845;
t939 = -t935;
t960 = t324+t725+t796;
t962 = t959.*1.08769e-2;
t967 = t959.*1.35652563578e-4;
t970 = t959.*7.0482312e-7;
t976 = t5.*t975;
t977 = t10.*t975;
t979 = t95+t298+t311+t694+t847;
t981 = t94+t300+t307+t696+t846;
t985 = t104+t300+t309+t696+t846;
t1086 = t39.*t1085;
t1095 = t137+t380+t384+t490+t594+t615+t617+t713+t755+t870;
t431 = -t427;
t495 = -t492;
t496 = -t494;
t529 = -t524;
t536 = -t528;
t537 = -t532;
t641 = t585.*(-7.0482312e-7);
t664 = t585.*(-4.0082304082032e-9);
t671 = t585.*(-2.261852897508832e-6);
t716 = t370+t587;
t721 = -t718;
t733 = dq6.*t715.*7.26350557185e-5;
t734 = t426+t605;
t743 = dq6.*t715.*1.745966317740249e-6;
t744 = dq6.*t715.*1.245668607194124e-6;
t748 = -t747;
t749 = t491+t639;
t750 = t493+t642;
t786 = t523+t663;
t808 = t582.*t685;
t812 = t582.*t687;
t813 = -t688.*(t234-t348);
t818 = t583.*t707;
t819 = t583.*t708;
t824 = t338+t340+t472+t483;
t826 = -t825;
t834 = -t832;
t837 = t108+t179+t402+t437+t554;
t848 = t390+t429+t517+t543;
t849 = t391+t428+t505+t544;
t853 = t99+t585+t742;
t856 = -t583.*(t524+t6.*(t234-t348).*4.203395243364607e-6);
t867 = t6.*t854.*4.36041e-5;
t868 = t11.*t854.*4.36041e-5;
t877 = t5.*t875;
t879 = t10.*t875;
t885 = -t882;
t886 = -t884;
t888 = t11.*(t90-t585+t10.*(dq4.*(t50+t239)+dq3.*t50.*5.110348748545983e-1+t4.*(t294-t295))).*(-1.33637554986e-4);
t889 = t6.*(t90-t585+t10.*(dq4.*(t50+t239)+dq3.*t50.*5.110348748545983e-1+t4.*(t294-t295))).*(-7.26350557185e-5);
t890 = t6.*(t90-t585+t10.*(dq4.*(t50+t239)+dq3.*t50.*5.110348748545983e-1+t4.*(t294-t295))).*7.26350557185e-5;
t891 = t11.*t854.*4.35810334311e-7;
t893 = t6.*t854.*8.01825329916e-7;
t900 = -t896;
t901 = -t897;
t902 = -t899;
t904 = -t903;
t905 = t11.*(t90-t585+t10.*(dq4.*(t50+t239)+dq3.*t50.*5.110348748545983e-1+t4.*(t294-t295))).*(-3.387428925624357e-6);
t906 = t6.*(t90-t585+t10.*(dq4.*(t50+t239)+dq3.*t50.*5.110348748545983e-1+t4.*(t294-t295))).*(-1.745966317740249e-6);
t907 = t6.*(t90-t585+t10.*(dq4.*(t50+t239)+dq3.*t50.*5.110348748545983e-1+t4.*(t294-t295))).*(-1.245668607194124e-6);
t908 = t11.*(t90-t585+t10.*(dq4.*(t50+t239)+dq3.*t50.*5.110348748545983e-1+t4.*(t294-t295))).*(-1.245668607194124e-6);
t909 = t6.*(t90-t585+t10.*(dq4.*(t50+t239)+dq3.*t50.*5.110348748545983e-1+t4.*(t294-t295))).*1.745966317740249e-6;
t910 = t6.*(t90-t585+t10.*(dq4.*(t50+t239)+dq3.*t50.*5.110348748545983e-1+t4.*(t294-t295))).*1.245668607194124e-6;
t911 = t715.*t730;
t912 = t715.*t731;
t913 = -t730.*(t368+t6.*(t234-t348));
t915 = -t729.*(t368+t6.*(t234-t348));
t916 = t729.*(t368+t6.*(t234-t348));
t917 = t349.*t833;
t919 = t582.*t816;
t920 = -t817.*(t234-t348);
t921 = t817.*(t234-t348);
t922 = t349.*t839;
t927 = -t926;
t929 = -t715.*(t492+t6.*(t234-t348).*1.33637554986e-4);
t931 = (t368+t6.*(t234-t348)).*(t494+t6.*(t234-t348).*7.26350557185e-5);
t932 = t715.*(t492+t6.*(t234-t348).*1.33637554986e-4);
t934 = t349.*t850;
t940 = -t936;
t941 = -t830.*(t234-t348);
t943 = -t836.*(t234-t348);
t945 = t582.*t840;
t947 = t467.*t875;
t948 = -t875.*(t91-t301);
t953 = t561.*t875;
t955 = t570.*t875;
t964 = -t962;
t969 = -t967;
t972 = -t970;
t973 = -t583.*(t492-t493+t6.*(t234-t348).*1.33637554986e-4+t11.*(t234-t348).*7.26350557185e-5);
t974 = t738.*t875;
t980 = dq4.*t979;
t982 = t5.*t979;
t983 = t10.*t979;
t984 = dq4.*t981;
t987 = t6.*t985;
t988 = t11.*t985;
t989 = t30.*t979;
t993 = t30.*t981;
et1 = t528-t531+t6.*(t234-t348).*3.387428925624357e-6;
et2 = t11.*(t234-t348).*1.245668607194124e-6;
t995 = -t715.*(et1+et2);
t996 = t59.*t979;
et3 = -t530+t532+t6.*(t234-t348).*1.245668607194124e-6;
et4 = t11.*(t234-t348).*1.745966317740249e-6;
t999 = (et3+et4).*(t368+t6.*(t234-t348));
t1001 = t59.*t981;
t1002 = t62.*t981;
t1003 = t67.*t979;
t1006 = t389.*t979;
t1007 = t389.*t981;
t1008 = -t979.*(t91-t301);
t1009 = t467.*t981;
t1010 = t979.*(t91-t301);
t1011 = t562.*t979;
t1012 = t563.*t979;
t1014 = -t981.*(t134-t350);
t1015 = t981.*(t134-t350);
t1016 = -t981.*(t149-t364);
t1017 = t981.*(t149-t364);
t1018 = t598.*t985;
t1019 = t599.*t985;
t1020 = t631.*t985;
t1021 = -t985.*(t302-t407);
t1023 = t326+t331+t851+t852;
t1032 = t732.*t979;
t1042 = t736.*t981;
t1046 = t324+t864+t977;
t1087 = -t1086;
t1094 = t130+t383+t385+t482+t597+t612+t618+t712+t753+t871;
t1133 = t242+t449+t452+t499+t503+t578+t728+t874+t880+t937+t938;
t735 = t431+t604;
t751 = t495+t638;
t752 = t496+t640;
t789 = t529+t662;
h = ft_2({dq1,dq2,dq3,dq4,dq5,dq6,t10,t1001,t1002,t1003,t1006,t1007,t1009,t1010,t1011,t1012,t1014,t1015,t1017,t1018,t1019,t1020,t1021,t1023,t1032,t1042,t1046,t1087,t109,t1094,t1095,t11,t111,t112,t1133,t114,t117,t12,t131,t138,t14,t146,t156,t157,t160,t167,t173,t174,t175,t176,t177,t181,t182,t183,t184,t185,t186,t189,t190,t191,t192,t193,t194,t195,t196,t197,t198,t199,t2,t201,t212,t231,t233,t234,t239,t241,t244,t245,t246,t247,t250,t251,t252,t254,t255,t256,t258,t259,t260,t261,t262,t263,t265,t266,t267,t268,t270,t271,t272,t274,t277,t282,t284,t294,t295,t3,t301,t302,t31,t323,t33,t337,t34,t343,t348,t349,t368,t371,t377,t379,t387,t388,t39,t4,t40,t407,t414,t419,t420,t422,t423,t427,t450,t455,t460,t461,t464,t466,t468,t471,t473,t475,t479,t480,t481,t485,t486,t489,t49,t492,t493,t494,t497,t498,t5,t50,t502,t504,t507,t509,t515,t518,t525,t526,t528,t53,t530,t531,t534,t535,t536,t537,t539,t540,t541,t547,t548,t549,t550,t553,t556,t569,t57,t577,t578,t579,t58,t582,t583,t585,t589,t59,t590,t591,t595,t6,t60,t600,t602,t603,t61,t610,t613,t619,t620,t621,t623,t624,t625,t626,t627,t628,t629,t63,t630,t631,t632,t633,t637,t64,t641,t643,t645,t647,t648,t649,t65,t650,t651,t652,t654,t656,t657,t658,t66,t660,t661,t664,t665,t666,t667,t668,t669,t671,t673,t674,t675,t679,t681,t682,t684,t685,t687,t688,t689,t692,t693,t697,t698,t699,t7,t703,t704,t705,t707,t708,t71,t710,t714,t715,t719,t72,t720,t721,t722,t723,t726,t727,t73,t733,t734,t737,t739,t74,t743,t744,t745,t746,t747,t748,t749,t75,t750,t751,t756,t757,t758,t759,t76,t760,t762,t763,t764,t765,t766,t768,t769,t77,t770,t771,t772,t773,t774,t775,t776,t777,t778,t78,t780,t781,t782,t783,t785,t786,t788,t790,t791,t792,t794,t795,t8,t80,t800,t805,t808,t810,t811,t812,t813,t814,t815,t816,t817,t818,t819,t820,t821,t823,t824,t826,t827,t828,t83,t831,t834,t835,t837,t838,t841,t842,t844,t845,t848,t849,t856,t857,t858,t860,t861,t862,t863,t866,t867,t868,t873,t875,t877,t878,t879,t882,t883,t884,t885,t886,t888,t890,t891,t893,t895,t896,t898,t9,t90,t900,t901,t902,t903,t904,t905,t908,t909,t91,t910,t911,t912,t913,t916,t917,t919,t921,t922,t925,t927,t931,t932,t934,t935,t936,t937,t938,t939,t940,t941,t943,t945,t947,t948,t953,t955,t958,t959,t960,t961,t963,t964,t965,t966,t968,t969,t971,t972,t973,t974,t975,t976,t978,t980,t982,t983,t984,t985,t987,t988,t993,t995,t996,t999});
end
function h = ft_2(ct)
dq1 = ct{1};
dq2 = ct{2};
dq3 = ct{3};
dq4 = ct{4};
dq5 = ct{5};
dq6 = ct{6};
t10 = ct{7};
t1001 = ct{8};
t1002 = ct{9};
t1003 = ct{10};
t1006 = ct{11};
t1007 = ct{12};
t1009 = ct{13};
t1010 = ct{14};
t1011 = ct{15};
t1012 = ct{16};
t1014 = ct{17};
t1015 = ct{18};
t1017 = ct{19};
t1018 = ct{20};
t1019 = ct{21};
t1020 = ct{22};
t1021 = ct{23};
t1023 = ct{24};
t1032 = ct{25};
t1042 = ct{26};
t1046 = ct{27};
t1087 = ct{28};
t109 = ct{29};
t1094 = ct{30};
t1095 = ct{31};
t11 = ct{32};
t111 = ct{33};
t112 = ct{34};
t1133 = ct{35};
t114 = ct{36};
t117 = ct{37};
t12 = ct{38};
t131 = ct{39};
t138 = ct{40};
t14 = ct{41};
t146 = ct{42};
t156 = ct{43};
t157 = ct{44};
t160 = ct{45};
t167 = ct{46};
t173 = ct{47};
t174 = ct{48};
t175 = ct{49};
t176 = ct{50};
t177 = ct{51};
t181 = ct{52};
t182 = ct{53};
t183 = ct{54};
t184 = ct{55};
t185 = ct{56};
t186 = ct{57};
t189 = ct{58};
t190 = ct{59};
t191 = ct{60};
t192 = ct{61};
t193 = ct{62};
t194 = ct{63};
t195 = ct{64};
t196 = ct{65};
t197 = ct{66};
t198 = ct{67};
t199 = ct{68};
t2 = ct{69};
t201 = ct{70};
t212 = ct{71};
t231 = ct{72};
t233 = ct{73};
t234 = ct{74};
t239 = ct{75};
t241 = ct{76};
t244 = ct{77};
t245 = ct{78};
t246 = ct{79};
t247 = ct{80};
t250 = ct{81};
t251 = ct{82};
t252 = ct{83};
t254 = ct{84};
t255 = ct{85};
t256 = ct{86};
t258 = ct{87};
t259 = ct{88};
t260 = ct{89};
t261 = ct{90};
t262 = ct{91};
t263 = ct{92};
t265 = ct{93};
t266 = ct{94};
t267 = ct{95};
t268 = ct{96};
t270 = ct{97};
t271 = ct{98};
t272 = ct{99};
t274 = ct{100};
t277 = ct{101};
t282 = ct{102};
t284 = ct{103};
t294 = ct{104};
t295 = ct{105};
t3 = ct{106};
t301 = ct{107};
t302 = ct{108};
t31 = ct{109};
t323 = ct{110};
t33 = ct{111};
t337 = ct{112};
t34 = ct{113};
t343 = ct{114};
t348 = ct{115};
t349 = ct{116};
t368 = ct{117};
t371 = ct{118};
t377 = ct{119};
t379 = ct{120};
t387 = ct{121};
t388 = ct{122};
t39 = ct{123};
t4 = ct{124};
t40 = ct{125};
t407 = ct{126};
t414 = ct{127};
t419 = ct{128};
t420 = ct{129};
t422 = ct{130};
t423 = ct{131};
t427 = ct{132};
t450 = ct{133};
t455 = ct{134};
t460 = ct{135};
t461 = ct{136};
t464 = ct{137};
t466 = ct{138};
t468 = ct{139};
t471 = ct{140};
t473 = ct{141};
t475 = ct{142};
t479 = ct{143};
t480 = ct{144};
t481 = ct{145};
t485 = ct{146};
t486 = ct{147};
t489 = ct{148};
t49 = ct{149};
t492 = ct{150};
t493 = ct{151};
t494 = ct{152};
t497 = ct{153};
t498 = ct{154};
t5 = ct{155};
t50 = ct{156};
t502 = ct{157};
t504 = ct{158};
t507 = ct{159};
t509 = ct{160};
t515 = ct{161};
t518 = ct{162};
t525 = ct{163};
t526 = ct{164};
t528 = ct{165};
t53 = ct{166};
t530 = ct{167};
t531 = ct{168};
t534 = ct{169};
t535 = ct{170};
t536 = ct{171};
t537 = ct{172};
t539 = ct{173};
t540 = ct{174};
t541 = ct{175};
t547 = ct{176};
t548 = ct{177};
t549 = ct{178};
t550 = ct{179};
t553 = ct{180};
t556 = ct{181};
t569 = ct{182};
t57 = ct{183};
t577 = ct{184};
t578 = ct{185};
t579 = ct{186};
t58 = ct{187};
t582 = ct{188};
t583 = ct{189};
t585 = ct{190};
t589 = ct{191};
t59 = ct{192};
t590 = ct{193};
t591 = ct{194};
t595 = ct{195};
t6 = ct{196};
t60 = ct{197};
t600 = ct{198};
t602 = ct{199};
t603 = ct{200};
t61 = ct{201};
t610 = ct{202};
t613 = ct{203};
t619 = ct{204};
t620 = ct{205};
t621 = ct{206};
t623 = ct{207};
t624 = ct{208};
t625 = ct{209};
t626 = ct{210};
t627 = ct{211};
t628 = ct{212};
t629 = ct{213};
t63 = ct{214};
t630 = ct{215};
t631 = ct{216};
t632 = ct{217};
t633 = ct{218};
t637 = ct{219};
t64 = ct{220};
t641 = ct{221};
t643 = ct{222};
t645 = ct{223};
t647 = ct{224};
t648 = ct{225};
t649 = ct{226};
t65 = ct{227};
t650 = ct{228};
t651 = ct{229};
t652 = ct{230};
t654 = ct{231};
t656 = ct{232};
t657 = ct{233};
t658 = ct{234};
t66 = ct{235};
t660 = ct{236};
t661 = ct{237};
t664 = ct{238};
t665 = ct{239};
t666 = ct{240};
t667 = ct{241};
t668 = ct{242};
t669 = ct{243};
t671 = ct{244};
t673 = ct{245};
t674 = ct{246};
t675 = ct{247};
t679 = ct{248};
t681 = ct{249};
t682 = ct{250};
t684 = ct{251};
t685 = ct{252};
t687 = ct{253};
t688 = ct{254};
t689 = ct{255};
t692 = ct{256};
t693 = ct{257};
t697 = ct{258};
t698 = ct{259};
t699 = ct{260};
t7 = ct{261};
t703 = ct{262};
t704 = ct{263};
t705 = ct{264};
t707 = ct{265};
t708 = ct{266};
t71 = ct{267};
t710 = ct{268};
t714 = ct{269};
t715 = ct{270};
t719 = ct{271};
t72 = ct{272};
t720 = ct{273};
t721 = ct{274};
t722 = ct{275};
t723 = ct{276};
t726 = ct{277};
t727 = ct{278};
t73 = ct{279};
t733 = ct{280};
t734 = ct{281};
t737 = ct{282};
t739 = ct{283};
t74 = ct{284};
t743 = ct{285};
t744 = ct{286};
t745 = ct{287};
t746 = ct{288};
t747 = ct{289};
t748 = ct{290};
t749 = ct{291};
t75 = ct{292};
t750 = ct{293};
t751 = ct{294};
t756 = ct{295};
t757 = ct{296};
t758 = ct{297};
t759 = ct{298};
t76 = ct{299};
t760 = ct{300};
t762 = ct{301};
t763 = ct{302};
t764 = ct{303};
t765 = ct{304};
t766 = ct{305};
t768 = ct{306};
t769 = ct{307};
t77 = ct{308};
t770 = ct{309};
t771 = ct{310};
t772 = ct{311};
t773 = ct{312};
t774 = ct{313};
t775 = ct{314};
t776 = ct{315};
t777 = ct{316};
t778 = ct{317};
t78 = ct{318};
t780 = ct{319};
t781 = ct{320};
t782 = ct{321};
t783 = ct{322};
t785 = ct{323};
t786 = ct{324};
t788 = ct{325};
t790 = ct{326};
t791 = ct{327};
t792 = ct{328};
t794 = ct{329};
t795 = ct{330};
t8 = ct{331};
t80 = ct{332};
t800 = ct{333};
t805 = ct{334};
t808 = ct{335};
t810 = ct{336};
t811 = ct{337};
t812 = ct{338};
t813 = ct{339};
t814 = ct{340};
t815 = ct{341};
t816 = ct{342};
t817 = ct{343};
t818 = ct{344};
t819 = ct{345};
t820 = ct{346};
t821 = ct{347};
t823 = ct{348};
t824 = ct{349};
t826 = ct{350};
t827 = ct{351};
t828 = ct{352};
t83 = ct{353};
t831 = ct{354};
t834 = ct{355};
t835 = ct{356};
t837 = ct{357};
t838 = ct{358};
t841 = ct{359};
t842 = ct{360};
t844 = ct{361};
t845 = ct{362};
t848 = ct{363};
t849 = ct{364};
t856 = ct{365};
t857 = ct{366};
t858 = ct{367};
t860 = ct{368};
t861 = ct{369};
t862 = ct{370};
t863 = ct{371};
t866 = ct{372};
t867 = ct{373};
t868 = ct{374};
t873 = ct{375};
t875 = ct{376};
t877 = ct{377};
t878 = ct{378};
t879 = ct{379};
t882 = ct{380};
t883 = ct{381};
t884 = ct{382};
t885 = ct{383};
t886 = ct{384};
t888 = ct{385};
t890 = ct{386};
t891 = ct{387};
t893 = ct{388};
t895 = ct{389};
t896 = ct{390};
t898 = ct{391};
t9 = ct{392};
t90 = ct{393};
t900 = ct{394};
t901 = ct{395};
t902 = ct{396};
t903 = ct{397};
t904 = ct{398};
t905 = ct{399};
t908 = ct{400};
t909 = ct{401};
t91 = ct{402};
t910 = ct{403};
t911 = ct{404};
t912 = ct{405};
t913 = ct{406};
t916 = ct{407};
t917 = ct{408};
t919 = ct{409};
t921 = ct{410};
t922 = ct{411};
t925 = ct{412};
t927 = ct{413};
t931 = ct{414};
t932 = ct{415};
t934 = ct{416};
t935 = ct{417};
t936 = ct{418};
t937 = ct{419};
t938 = ct{420};
t939 = ct{421};
t940 = ct{422};
t941 = ct{423};
t943 = ct{424};
t945 = ct{425};
t947 = ct{426};
t948 = ct{427};
t953 = ct{428};
t955 = ct{429};
t958 = ct{430};
t959 = ct{431};
t960 = ct{432};
t961 = ct{433};
t963 = ct{434};
t964 = ct{435};
t965 = ct{436};
t966 = ct{437};
t968 = ct{438};
t969 = ct{439};
t971 = ct{440};
t972 = ct{441};
t973 = ct{442};
t974 = ct{443};
t975 = ct{444};
t976 = ct{445};
t978 = ct{446};
t980 = ct{447};
t982 = ct{448};
t983 = ct{449};
t984 = ct{450};
t985 = ct{451};
t987 = ct{452};
t988 = ct{453};
t993 = ct{454};
t995 = ct{455};
t996 = ct{456};
t999 = ct{457};
t809 = -t808;
t855 = t583.*t786;
t869 = -t868;
t881 = -t879;
t887 = t349.*t824;
t892 = -t891;
t894 = -t893;
t914 = -t912;
t918 = -t917;
t923 = -t922;
t928 = t715.*t749;
t930 = -t750.*(t368+t6.*(t234-t348));
t933 = t750.*(t368+t6.*(t234-t348));
t942 = t582.*t837;
t946 = -t945;
t949 = t582.*t849;
t950 = -t848.*(t234-t348);
t952 = t848.*(t234-t348);
t954 = -t953;
t956 = t531+t536+t665+t668;
t957 = t530+t537+t666+t667;
t986 = -t982;
t990 = t980.*1.08769e-2;
t991 = t980.*(-2.889644e-2);
t994 = t984.*(-2.889644e-2);
t997 = t980.*1.35652563578e-4;
t998 = t980.*6.1855407534e-5;
t1004 = -t999;
t1005 = t980.*(-1.869599668e-7);
t1013 = -t1011;
t1022 = -t1020;
t1024 = t9.*t1023;
t1025 = t4.*t1023;
t1038 = -t1032;
t1043 = -t1042;
t1044 = t824.*t985;
t1047 = t423+t877+t983;
t1097 = t173+t377+t379+t556+t857+t858+t925+t927;
t1134 = t241+t450+t455+t498+t502+t579+t727+t873+t878+t939+t940;
t1135 = t31.*t40.*t1133.*9.543032792050485e-17;
t1138 = t182+t201+t387+t388+t485+t486+t497+t595+t625+t628+t703+t705+t714+t805+t1009+t1010;
t944 = t750+t751;
t951 = -t949;
t992 = -t990;
t1000 = -t998;
t1026 = t1025.*2.889644e-2;
t1027 = t1024.*2.889644e-2;
t1030 = t1024.*1.08769e-2;
t1033 = t1025.*1.688944904408e-4;
t1034 = t1024.*6.1855407534e-5;
t1035 = t1025.*6.678441185616e-4;
t1036 = t1024.*6.678441185616e-4;
t1037 = t1024.*1.35652563578e-4;
t1040 = t1024.*1.869599668e-7;
t1045 = -t1044;
t1048 = t414+t879+t986;
t1049 = t6.*t1047;
t1050 = t11.*t1047;
t1051 = -dq5.*(t422+t881+t982);
t1053 = dq5.*t1047.*7.26735e-3;
t1054 = t34.*t1047;
t1056 = -t34.*(t422+t881+t982);
t1057 = dq5.*t1047.*(-1.08769e-2);
t1058 = dq5.*(t422+t881+t982).*1.08769e-2;
t1059 = dq5.*t1047.*7.26350557185e-5;
t1060 = t58.*t1047;
t1061 = dq5.*t1047.*1.33637554986e-4;
t1063 = dq5.*t1047.*(-6.1855407534e-5);
t1064 = dq5.*(t422+t881+t982).*(-1.35652563578e-4);
t1066 = t65.*t1047;
t1067 = t60.*(t422+t881+t982);
t1068 = dq5.*(t422+t881+t982).*(-7.0482312e-7);
t1069 = dq5.*t1047.*(-7.0482312e-7);
t1070 = t65.*(t422+t881+t982);
t1071 = t14+t57+t244+t422+t881+t982;
t1072 = t539.*t1047;
t1073 = -t539.*(t422+t881+t982);
t1074 = t631.*t1047;
t1075 = (t302-t407).*(t422+t881+t982);
t1076 = -t1047.*(t337-t473);
t1077 = -t685.*(t422+t881+t982);
t1078 = t1047.*(t337-t473);
t1079 = -t687.*(t422+t881+t982);
t1080 = t688.*t1047;
t1081 = t687.*(t422+t881+t982);
t1088 = t817.*t1047;
t1089 = -t816.*(t422+t881+t982);
t1107 = t131+t600+t862+t984+t1025;
t1123 = t138+t419+t602+t860+t980+t1024;
t1136 = t31.*t40.*t1134.*5.673626844500105e-17;
t1137 = -t1135;
t1028 = -t1026;
t1029 = -t1027;
t1031 = -t1030;
t1039 = -t1034;
t1041 = -t1040;
t1052 = -t1050;
t1055 = -t1053;
t1062 = -t1059;
t1065 = -t1061;
t1082 = t707.*t1071;
t1083 = t708.*t1071;
t1090 = -t1088;
t1091 = t734.*t1071;
t1092 = -t1071.*(t427+t6.*(t234-t348).*7.26735e-3);
t1093 = t1071.*(t427+t6.*(t234-t348).*7.26735e-3);
t1096 = -t1071.*(t492-t493+t6.*(t234-t348).*1.33637554986e-4+t11.*(t234-t348).*7.26350557185e-5);
t1098 = t591+t988+t1049;
t1108 = t10.*t1107;
t1112 = t5.*t1107.*1.08769e-2;
t1114 = t5.*t1107.*7.26735e-3;
t1116 = t5.*t1107.*1.33637554986e-4;
t1117 = t5.*t1107.*7.26350557185e-5;
t1118 = t5.*t1107.*6.1855407534e-5;
t1120 = t5.*t1107.*7.0482312e-7;
t1128 = t11.*t1123.*7.26735e-3;
t1129 = t6.*t1123.*7.26735e-3;
t1131 = t6.*t1123.*1.33637554986e-4;
t1132 = t11.*t1123.*7.26350557185e-5;
t1147 = t259+t261+t262+t460+t461+t525+t535+t540+t610+t656+t657+t719+t823+t835+t838+t898+t955+t996+t1017+t1036+t1038;
t1148 = t245+t263+t277+t464+t466+t541+t547+t553+t613+t660+t675+t722+t826+t831+t834+t902+t954+t1001+t1012+t1035+t1043;
et5 = -t250-t265-t271-t343.*6.634286610512106e-7+t820-t827+t896+t903-t974-t984.*1.688944904408e-4;
et6 = t1003+t1011+t1014-t1033+t1040+t117.*(t50+t239)+t800.*(t50+t239)+t4.*(t294-t295).*8.487305697640184e-9;
et7 = t9.*(t294-t295).*4.427198467956924e-6;
t1156 = t31.*t40.*(et5+et6+et7).*(-9.543032792050485e-17);
t1084 = -t1083;
t1099 = t590+t987+t1052;
t1100 = t33.*t1098;
t1101 = dq6.*t1098.*(-7.26735e-3);
t1104 = t61.*t1098;
t1109 = -t1108;
t1110 = t669.*t1098;
t1113 = t1108.*1.08769e-2;
t1115 = t1108.*1.35652563578e-4;
t1119 = t1108.*7.0482312e-7;
t1121 = t734.*t1098;
t1124 = t750.*t1098;
t1125 = -t1098.*(t494+t6.*(t234-t348).*7.26350557185e-5);
t1130 = -t1129;
t1140 = t6.*(t747-t959+t1108+dq5.*(t422+t881+t982)).*(-7.26735e-3);
t1141 = t11.*(t747-t959+t1108+dq5.*(t422+t881+t982)).*(-7.26735e-3);
t1142 = t11.*(t747-t959+t1108+dq5.*(t422+t881+t982)).*(-1.33637554986e-4);
t1143 = t6.*(t747-t959+t1108+dq5.*(t422+t881+t982)).*(-7.26350557185e-5);
t1144 = t11.*(t747-t959+t1108+dq5.*(t422+t881+t982)).*1.33637554986e-4;
t1145 = t196+t198+t481+t619+t681+t704+t815+t885+t947+t991+t1006+t1029;
t1146 = t176+t197+t475+t623+t684+t710+t811+t883+t948+t994+t1007+t1028;
t1149 = t272.*t1147;
t1151 = t270.*t1148;
t1152 = t183+t192+t193+t479+t627+t629+t637+t762+t763+t812+t813+t886+t887+t992+t1031+t1074+t1075;
t1153 = t175+t194+t468+t624+t641+t720+t756+t768+t810+t919+t963+t1021+t1057+t1072+t1112;
t1155 = t250+t265+t271+t504+t534+t647+t654+t821+t827+t828+t900+t904+t974+t1002+t1005+t1013+t1015+t1033+t1041;
t1158 = t247+t252+t256+t267+t515+t518+t650+t651+t658+t671+t776+t782+t790+t895+t923+t941+t946+t971+t997+t1019+t1037+t1069+t1077+t1090+t1120;
t1102 = t33.*t1099;
t1103 = dq6.*t1099.*(-7.26735e-3);
t1105 = t63.*t1099;
t1106 = dq6.*t1099.*(-7.26350557185e-5);
t1111 = t669.*t1099;
t1122 = -t1099.*(t427+t6.*(t234-t348).*7.26735e-3);
t1126 = t749.*t1099;
t1127 = -t1099.*(t492+t6.*(t234-t348).*1.33637554986e-4);
t1139 = t748+t959+t1051+t1109;
t1150 = -t1149;
t1154 = t177+t195+t471+t621+t645+t721+t757+t766+t809+t921+t964+t1022+t1058+t1073+t1113;
t1159 = t255+t258+t266+t268+t509+t548+t649+t652+t673+t674+t777+t780+t788+t901+t918+t942+t943+t972+t1000+t1018+t1039+t1070+t1078+t1089+t1119;
t1160 = -t1158.*(t160-t284);
t1161 = t1158.*(t160-t284);
et8 = t255+t258+t266+t268+t509+t548+t585.*7.314371377091851e-7;
et9 = t589.*5.918087154269792e-7+t649+t674+t777+t780+t788+t901+t918+t942+t943+t972+t1000+t1018+t1039+t1078+t1089+t1119;
et10 = dq5.*(t422+t881+t982).*7.0482312e-7;
t1162 = t526.*(et8+et9+et10);
t1168 = t181+t643+t764+t818+t867+t931+t932+t1093+t1101+t1110+t1130+t1141;
t1170 = t254+t260+t274+t507+t648+t664+t679+t769+t771+t785+t792+t934+t951+t952+t966+t969+t1045+t1063+t1067+t1080+t1081+t1115+t1118;
t1157 = t146+t420+t603+t733+t737+t758+t759+t760+t888+t890+t961+t973+t1055+t1114+t1121+t1122;
t1163 = t186+t480+t626+t743+t745+t770+t773+t774+t855+t908+t909+t913+t914+t965+t1062+t1084+t1117+t1124+t1126;
t1164 = t199+t489+t630+t744+t746+t772+t775+t778+t856+t905+t910+t911+t916+t968+t1065+t1082+t1116+t1125+t1127;
t1165 = -(t282+t6.*(t160-t284)).*(t186+t480+t626+t770+t773+t774+t855+t908+t909+t913+t914+t965+t1062+t1084+t1117+t1124+t1126-t112.*(t368+t6.*(t234-t348))+t111.*t715);
t1166 = (t282+t6.*(t160-t284)).*(t186+t480+t626+t770+t773+t774+t855+t908+t909+t913+t914+t965+t1062+t1084+t1117+t1124+t1126-t112.*(t368+t6.*(t234-t348))+t111.*t715);
t1169 = t190+t632+t765+t819+t869+t928+t933+t1091+t1103+t1111+t1128+t1140;
t1171 = t270.*t1170;
t1172 = t251+t661+t783+t892+t894+t995+t1004+t1096+t1104+t1106+t1131+t1132+t1143+t1144;
et11 = t528-t531+t6.*(t234-t348).*3.387428925624357e-6;
et12 = t11.*(t234-t348).*1.245668607194124e-6;
et13 = t246+t589.*4.203395243364607e-6+t781+t891+t893+t999+t1105-t1131-t1132+t1142-dq6.*t1098.*1.33637554986e-4;
et14 = t6.*(t747-t959+t1108+dq5.*(t422+t881+t982)).*7.26350557185e-5+t715.*(et11+et12);
et15 = t1071.*(t492-t493+t6.*(t234-t348).*1.33637554986e-4+t11.*(t234-t348).*7.26350557185e-5);
t1173 = -t526.*(et13+et14+et15);
et16 = t528-t531+t6.*(t234-t348).*3.387428925624357e-6;
et17 = t11.*(t234-t348).*1.245668607194124e-6;
et18 = t246+t589.*4.203395243364607e-6+t781+t891+t893+t999+t1105-t1131-t1132+t1142-dq6.*t1098.*1.33637554986e-4;
et19 = t6.*(t747-t959+t1108+dq5.*(t422+t881+t982)).*7.26350557185e-5+t715.*(et16+et17);
et20 = t1071.*(t492-t493+t6.*(t234-t348).*1.33637554986e-4+t11.*(t234-t348).*7.26350557185e-5);
t1174 = t526.*(et18+et19+et20);
t1167 = t682.*t1164;
et21 = t77.*(-2.038587e-2)+t2.*t8.*1.999853847e-1+t3.*t7.*1.999853847e-1;
et22 = -t12.*(dq1.*4.573233567645e-4+dq2.*4.573233567645e-4)+dq1.*t64.*t71;
et23 = t83+t693+t842-t9.*t31.*t40.*2.479366200131245e-18;
et24 = -(t191-t196-t681-t704+t814+t882-t947+t980.*2.889644e-2-t1006+t1027+t59.*(t50+t239)+t4.*(t294-t295).*1.3117937708872e-3);
et25 = -t183+t184+t185-t585.*1.35652563578e-4+t633-t812+t884-t887+t990+t1030-t1074-t1075+dq4.*(t50+t239).*4.71413003675e-4;
et26 = t4.*(t294-t295).*7.13801892181e-4+t688.*(t234-t348);
et27 = t5.*(dq4.*(t50+t239)+dq3.*t50.*5.110348748545983e-1+t4.*(t294-t295)).*6.1855407534e-5;
et28 = t10.*(dq4.*(t50+t239)+dq3.*t50.*5.110348748545983e-1+t4.*(t294-t295)).*1.35652563578e-4;
et29 = t75.*(-2.038587e-2)-t2.*t3.*1.999853847e-1+t7.*t8.*1.999853847e-1;
et30 = t12.*(dq1.*3.222314966007e-4+dq2.*3.222314966007e-4)+dq1.*t64.*t66;
et31 = t2.*(-4.710919801360536e-3)-t7.*2.43593206408921e-2+t72+t73+t78+t80+t156+t157+t1087+t1136+t1137+t1150+t1151+t1156+t1161+t1162+t1166+t1167+t1171+t1174+t1168.*(t549+t6.*t978-t11.*t1046)-t1169.*(t550+t11.*t978+t6.*t1046)+t689.*t1097+t841.*t1094;
et32 = -t863.*t1138+t1046.*t1154+t975.*(t174+t189+t343.*6.678441185616e-4+t620-t684-t710-t811-t883+t993-t1007+t1026+t875.*(t91-t301))+t1157.*(t53+t167+t323+t866+t976)-t66.*(et21+et22)-t1095.*(t371+t569+t698)+t1153.*(t323+t866+t976)+et23.*et24-t978.*(et25+et26+et27+et28)+t71.*(et29+et30);
et33 = t83+t699-t9.*t31.*t40.*7.351481000981246e-18;
et34 = -(t191-t196-t681-t704+t814+t882-t947+t980.*2.889644e-2-t1006+t1027+t59.*(t50+t239)+t4.*(t294-t295).*1.3117937708872e-3);
et35 = -t183+t184+t185-t585.*1.35652563578e-4+t633-t812+t884-t887+t990+t1030-t1074-t1075+dq4.*(t50+t239).*4.71413003675e-4;
et36 = t4.*(t294-t295).*7.13801892181e-4+t688.*(t234-t348);
et37 = t5.*(dq4.*(t50+t239)+dq3.*t50.*5.110348748545983e-1+t4.*(t294-t295)).*6.1855407534e-5;
et38 = t10.*(dq4.*(t50+t239)+dq3.*t50.*5.110348748545983e-1+t4.*(t294-t295)).*1.35652563578e-4;
et39 = t9.*(t191-t196-t681-t704+t814+t882-t947+t980.*2.889644e-2-t1006+t1027+t59.*(t50+t239)+t4.*(t294-t295).*1.3117937708872e-3);
et40 = -1.264860527128474e-2;
et41 = t255+t258+t266+t268+t509+t548+t585.*7.314371377091851e-7;
et42 = t589.*5.918087154269792e-7+t649+t674+t777+t780+t788+t901+t918+t942+t943+t972+t1000+t1018+t1039+t1078+t1089+t1119;
et43 = dq5.*(t422+t881+t982).*7.0482312e-7;
et44 = t528-t531+t6.*(t234-t348).*3.387428925624357e-6;
et45 = t11.*(t234-t348).*1.245668607194124e-6;
et46 = t246+t589.*4.203395243364607e-6+t781+t891+t893+t999+t1105-t1131-t1132+t1142-dq6.*t1098.*1.33637554986e-4;
et47 = t6.*(t747-t959+t1108+dq5.*(t422+t881+t982)).*7.26350557185e-5+t715.*(et44+et45);
et48 = t1071.*(t492-t493+t6.*(t234-t348).*1.33637554986e-4+t11.*(t234-t348).*7.26350557185e-5);
et49 = -t183+t184+t185-t585.*1.35652563578e-4+t633-t812+t884-t887+t990+t1030-t1074-t1075+dq4.*(t50+t239).*4.71413003675e-4;
et50 = t4.*(t294-t295).*7.13801892181e-4+t688.*(t234-t348);
et51 = t5.*(dq4.*(t50+t239)+dq3.*t50.*5.110348748545983e-1+t4.*(t294-t295)).*6.1855407534e-5;
et52 = t10.*(dq4.*(t50+t239)+dq3.*t50.*5.110348748545983e-1+t4.*(t294-t295)).*1.35652563578e-4;
et53 = t343.*3.390351827752591e-7+t577.*8.595599785252598e-1;
et54 = t578.*(-5.110348748545983e-1)-t820.*5.110348748545983e-1+t827.*5.110348748545983e-1;
et55 = t860.*(-9.554306323645785e-8);
et56 = t861.*(-8.631097478604537e-5)+t935.*8.595599785252598e-1+t936.*8.595599785252598e-1;
et57 = t937.*(-5.110348748545983e-1)-t938.*5.110348748545983e-1+t974.*5.110348748545983e-1;
et58 = t980.*(-9.554306323645785e-8);
et59 = t984.*8.631097478604537e-5-t1011.*5.110348748545983e-1+t1015.*5.110348748545983e-1;
et60 = t1024.*(-9.554306323645785e-8);
et61 = t1025.*8.631097478604537e-5;
et62 = dq4.*(t50+t239).*(-2.208156882018249e-9)+et39.*et40-t800.*(t50+t239).*5.110348748545983e-1;
et63 = dq3.*t49.*2.100768039879952e-6;
et64 = dq3.*t50.*(-3.26212675506904e-9);
et65 = dq3.*t844.*(-4.586198809426854e-6);
et66 = dq3.*t845.*(-7.713980286110893e-6);
et67 = -t1157.*(t4.*5.157359871151559e-3+t4.*t5.*4.990257941055339e-2)-t4.*t1148.*8.595599785252598e-1-t9.*t1147.*8.595599785252598e-1;
et68 = t4.*t1170.*(-8.595599785252598e-1)+t76.*t1158+t74.*(et41+et42+et43);
et69 = t4.*(t174+t189+t343.*6.678441185616e-4+t620-t684-t710-t811-t883+t993-t1007+t1026+t875.*(t91-t301)).*(-1.264860527128474e-2);
et70 = t4.*(t294-t295).*(-4.33730920504627e-9);
et71 = t9.*(t294-t295).*(-2.262452815028836e-6)+t74.*(et46+et47+et48);
et72 = t9.*(et49+et50+et51+et52).*(-4.990257941055339e-2)-t1164.*(t4.*t6.*8.595599785252598e-1+t11.*t76);
et73 = -(t4.*t11.*8.595599785252598e-1-t6.*t76).*(t186+t480+t626+t770+t773+t774+t855+t908+t909+t913+t914+t965+t1062+t1084+t1117+t1124+t1126-t112.*(t368+t6.*(t234-t348))+t111.*t715);
et74 = t1168.*(t6.*t9.*4.990257941055339e-2+t6.*t74.*(3.0./5.0e+2)+t4.*t10.*t11.*4.990257941055339e-2);
et75 = -t1169.*(t9.*t11.*4.990257941055339e-2+t11.*t74.*(3.0./5.0e+2)-t4.*t6.*t10.*4.990257941055339e-2);
et76 = dq3.*t12.*t39.*1.680244941984175e-6;
et77 = t31.*t40.*t109.*(-8.564238525144865e-22);
et78 = t31.*t40.*t114.*5.091703513734173e-22;
et79 = t12.*t39.*t231.*(-5.321009981904056e-7);
et80 = t12.*t39.*t233.*4.553682647545594e-7;
et81 = t12.*t39.*t692.*(-4.515804245053758e-5)-t4.*t5.*t1153.*4.990257941055339e-2;
et82 = t4.*t10.*t1154.*(-4.990257941055339e-2);
et83 = t255+t258+t266+t268+t509+t548+t585.*7.314371377091851e-7;
et84 = t589.*5.918087154269792e-7+t649+t674+t777+t780+t788+t901+t918+t942+t943+t972+t1000+t1018+t1039+t1078+t1089+t1119;
et85 = dq5.*(t422+t881+t982).*7.0482312e-7;
et86 = t528-t531+t6.*(t234-t348).*3.387428925624357e-6;
et87 = t11.*(t234-t348).*1.245668607194124e-6;
et88 = t246+t589.*4.203395243364607e-6+t781+t891+t893+t999+t1105-t1131-t1132+t1142-dq6.*t1098.*1.33637554986e-4;
et89 = t6.*(t747-t959+t1108+dq5.*(t422+t881+t982)).*7.26350557185e-5+t715.*(et86+et87);
et90 = t1071.*(t492-t493+t6.*(t234-t348).*1.33637554986e-4+t11.*(t234-t348).*7.26350557185e-5);
et91 = t260+t274+t343.*2.925194867859459e-6+t664+t679+t771+t785+t792+t934+t951+t952+t969+t1045+t1067+t1080+t1081+t1115+t1121.*(3.0./5.0e+2);
et92 = dq6.*(t368+t6.*(t234-t348)).*(-8.01825329916e-7);
et93 = dq3.*t49.*1.494876593221872e-6;
et94 = dq6.*t715.*4.35810334311e-7-dq5.*t1047.*1.05459507534e-4;
et95 = t5.*t739.*4.57069415115421e-6+t6.*t739.*8.01825329916e-7;
et96 = t11.*t739.*4.35810334311e-7+t10.*t958.*1.05459507534e-4;
et97 = t5.*t1107.*1.05459507534e-4+t6.*t1164+t11.*(t186+t480+t626+t770+t773+t774+t855+t908+t909+t913+t914+t965+t1062+t1084+t1117+t1124+t1126-t112.*(t368+t6.*(t234-t348))+t111.*t715);
et98 = t6.*(t90-t585+t10.*(dq4.*(t50+t239)+dq3.*t50.*5.110348748545983e-1+t4.*(t294-t295))).*4.35810334311e-7;
et99 = t11.*(t90-t585+t10.*(dq4.*(t50+t239)+dq3.*t50.*5.110348748545983e-1+t4.*(t294-t295))).*(-8.01825329916e-7);
et100 = t9.*(t294-t295).*(-2.925194867859459e-6);
et101 = t583.*(t492-t493+t6.*(t234-t348).*1.33637554986e-4+t11.*(t234-t348).*7.26350557185e-5).*(-3.0./5.0e+2);
et102 = t1099.*(t427+t6.*(t234-t348).*7.26735e-3).*(-3.0./5.0e+2);
et103 = t528-t531+t6.*(t234-t348).*3.387428925624357e-6;
et104 = t11.*(t234-t348).*1.245668607194124e-6;
et105 = t246+t589.*4.203395243364607e-6+t781+t891+t893+t999+t1105-t1131-t1132+t1142-dq6.*t1098.*1.33637554986e-4;
et106 = t6.*(t747-t959+t1108+dq5.*(t422+t881+t982)).*7.26350557185e-5+t715.*(et103+et104);
et107 = t1071.*(t492-t493+t6.*(t234-t348).*1.33637554986e-4+t11.*(t234-t348).*7.26350557185e-5);
mt1 = [et31+et32,t72+t73+t78+t80+t156+t157+t1087+t1136+t1137+t1150+t1151+t1156+t1161+t1162+t1166+t1167+t1171+t1174+et33.*et34+t1168.*(t549+t6.*t794-t11.*t960)-t1169.*(t550+t11.*t794+t6.*t960)+t212.*t1097+t697.*t1094-t698.*t1095-t723.*t1138+t960.*t1154+t791.*(t174+t189+t343.*6.678441185616e-4+t620-t684-t710-t811-t883+t993-t1007+t1026+t875.*(t91-t301))+t1157.*(t53+t167+t323+t726+t795)+t1153.*(t323+t726+t795)-t794.*(et35+et36+et37+et38)];
mt2 = [et53+et54+et55+et56+et57+et58+et59+et60+et61+et62+et63+et64+et65+et66+et67+et68+et69+et70+et71+et72+et73+et74+et75+et76+et77+et78+et79+et80+et81+et82,t1155+t5.*t1158+t10.*(et83+et84+et85)+t10.*(et88+et89+et90)-t5.*t11.*t1164+t6.*t10.*t1168.*(3.0./5.0e+2)-t10.*t11.*t1169.*(3.0./5.0e+2)+t5.*t6.*(t186+t480+t626+t770+t773+t774+t855+t908+t909+t913+t914+t965+t1062+t1084+t1117+t1124+t1126-t112.*(t368+t6.*(t234-t348))+t111.*t715),et91+et92+et93+et94+et95+et96+et97+et98+et99+et100+et101+et102,et105+et106+et107];
h = real(reshape([mt1,mt2],6,1));
end
